simulink model "Control_Model"  (R2015a)
settings: Solver=ode1  StartTime=0.0  StopTime=150  FixedStep=0.002  MaxStep=0.01  MinStep=0.01  RelTol=1e-3
settings Model: Creator=Callum  LastModifiedBy=Callum
settings SolverCC: InitialStep=0.01
settings HardwareCC: TargetLongLongMode=on  TargetIntDivRoundTo=Zero  TargetEndianess=LittleEndian  TargetHWDeviceType=MATLAB Host  ProdEqTarget=off
settings RTWCC: SystemTargetFile=rsim.tlc  TemplateMakefile=rsim_default_tmf  Description=Rapid Simulation Target
settings RSimTargetCC: ERTMultiwordTypeDef=System defined  ERTMultiwordLength=256

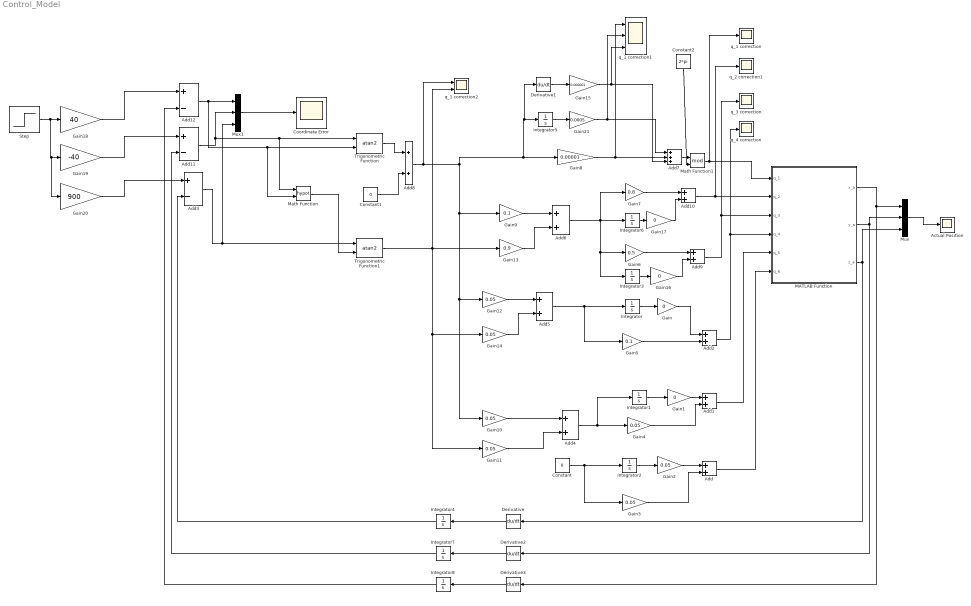
== system Control_Model ==
  Actual Position : Scope
      settings: YMin=-400  YMax=1200
  Add{,1..2,4..6,8..10} (9 alike) : Sum
  Add11 : Sum  Inputs=+-
  Add12 : Sum  Inputs=+-
  Add3 : Sum  Inputs=+-
  Add7 : Sum  Inputs=+++
  Constant : Constant  Value=0
  Constant1 : Constant  Value=0
  Constant2 : Constant  Value=2*pi
  Coordinate Error : Scope
      settings: SaveName=ScopeData7
  Derivative{,1..3} (4 alike) : Derivative
  Gain{,1,16..17} (4 alike) : Gain  Gain=0
  Gain{2..4,10..12,14} (7 alike) : Gain  Gain=0.05
  Gain13 : Gain  Gain=0.9
  Gain15 : Gain  Gain=0.000001
  Gain18 : Gain  Gain=40
  Gain19 : Gain  Gain=-40
  Gain20 : Gain  Gain=900
  Gain21 : Gain  Gain=0.0005
  Gain5 : Gain  Gain=0.1
  Gain6 : Gain  Gain=0.5
  Gain7 : Gain  Gain=0.8
  Gain8 : Gain  Gain=0.00001
  Gain9 : Gain  Gain=0.1
  Integrator{,1..8} (9 alike) : Integrator
  MATLAB Function : MATLAB Function  TreatAsAtomicUnit=on
  Math Function : Math  Operator=hypot  SaturateOnIntegerOverflow=on
  Math Function1 : Math  Operator=mod  SaturateOnIntegerOverflow=on
  Mux : Mux  Inputs=3
  Mux1 : Mux  Inputs=3
  Step : Step  SampleTime=0
  Trigonometric Function : Trigonometry  Operator=atan2
  Trigonometric Function1 : Trigonometry  Operator=atan2
  q_1 correction : Scope
      settings: YMin=0  YMax=6.5
  q_1 correction1 : Scope  NumInputPorts=3
      settings: YMin=-5~-5~-5  YMax=5~5~5  SaveName=ScopeData5
  q_1 correction2 : Scope  NumInputPorts=2
      settings: YMin=-5~-5  YMax=5~5  SaveName=ScopeData6
  q_2 correction1 : Scope
      settings: SaveName=ScopeData2
  q_3 correction : Scope
      settings: SaveName=ScopeData3
  q_4 correction : Scope
      settings: SaveName=ScopeData4
  wires:
  Integrator/1 -> Gain/1
  Integrator1/1 -> Gain1/1
  Integrator2/1 -> Gain2/1
  Constant/1 -> Integrator2/1, Gain3/1
  Gain2/1 -> Add/1
  Gain3/1 -> Add/2
  Add/1 -> MATLAB Function/6(q_6)
  Gain1/1 -> Add1/1
  Add1/1 -> MATLAB Function/5(q_5)
  Gain4/1 -> Add1/2
  Add2/1 -> q_4 correction/1, MATLAB Function/4(q_4)
  Gain/1 -> Add2/1
  Gain5/1 -> Add2/2
  Add4/1 -> Integrator1/1, Gain4/1
  Add5/1 -> Gain5/1, Integrator/1
  Add6/1 -> Gain6/1, Integrator3/1, Integrator6/1, Gain7/1
  Gain18/1 -> Add12/1
  Gain20/1 -> Add3/1
  Add11/1 -> Mux1/2, Math Function/1, Trigonometric Function/1
  MATLAB Function/1(x_a) -> Mux/1, Derivative3/1
  MATLAB Function/3(z_a) -> Mux/3, Derivative/1
  Gain10/1 -> Add4/1
  Gain11/1 -> Add4/2
  Gain14/1 -> Add5/2
  Add12/1 -> Mux1/1, Trigonometric Function/2, Math Function/2
  Step/1 -> Gain20/1, Gain19/1, Gain18/1
  Gain19/1 -> Add11/1
  Gain6/1 -> Add9/1
  Integrator4/1 -> Add3/2
  Derivative/1 -> Integrator4/1
  Integrator5/1 -> Gain21/1
  Gain21/1 -> q_1 correction1/2, Add7/1
  Add7/1 -> Math Function1/1
  Gain8/1 -> q_1 correction1/1, Add7/2
  Trigonometric Function/1 -> Add8/1
  Constant1/1 -> Add8/2
  Add8/1 -> q_1 correction2/1, Gain9/1, Gain10/1, Gain12/1, Derivative1/1, Integrator5/1, Gain8/1
  Gain12/1 -> Add5/1
  Gain13/1 -> Add6/2
  Gain9/1 -> Add6/1
  Trigonometric Function1/1 -> Gain13/1, q_1 correction2/2, Gain11/1, Gain14/1
  Add3/1 -> Mux1/3, Trigonometric Function1/1
  Math Function/1 -> Trigonometric Function1/2
  Derivative1/1 -> Gain15/1
  Gain15/1 -> q_1 correction1/3, Add7/3
  Math Function1/1 -> q_1 correction/1, MATLAB Function/1(q_1)
  Constant2/1 -> Math Function1/2
  Integrator3/1 -> Gain16/1
  Gain16/1 -> Add9/2
  Add9/1 -> q_3 correction/1, MATLAB Function/3(q_3)
  Integrator6/1 -> Gain17/1
  Gain7/1 -> Add10/1
  Gain17/1 -> Add10/2
  Add10/1 -> MATLAB Function/2(q_2), q_2 correction1/1
  MATLAB Function/2(y_a) -> Derivative2/1, Mux/2
  Integrator7/1 -> Add11/2
  Derivative2/1 -> Integrator7/1
  Derivative3/1 -> Integrator8/1
  Integrator8/1 -> Add12/2
  Mux/1 -> Actual Position/1
  Mux1/1 -> Coordinate Error/1

== matlab function Control_Model/MATLAB Function ==
  data: q_1 input; x_a output; q_2 input; q_3 input; q_4 input; q_5 input; q_6 input; y_a output; z_a output
function [x_a, y_a, z_a] = fcn(q_1, q_2, q_3, q_4, q_5, q_6)
%#codegen

q1 = q_1; %pi-(q_1);
q2 = q_2; %-pi/2 + (q_2+pi);
q3 = q_3; %pi/2 + (pi+q_3);
q4 = q_4; %q_4;
q5 = q_5; %-pi + q_5;
q6 = q_6; %pi + q_6;

%A_new = vpa(subs(A, [q1,q2,q3,q4,q5,q6], [ pi-(q_1), -pi/2 + (q_2+pi), pi/2 + (pi+q_3), q_4, -pi + q_5, pi]));


x_a = 9.8*sin(q1) + 410.0*cos(q1)*cos(q2) - 161.90703230275506147226218323136*cos(q4)*sin(q1) + 175.614064605510166451876962007*sin(q5)*(1.0*sin(q1)*sin(q4) - cos(q4)*(cos(q1)*cos(q2)*cos(q3) + cos(q1)*sin(q2)*sin(q3))) - 161.90703230275506147226218323136*sin(q4)*(cos(q1)*cos(q2)*cos(q3) + cos(q1)*sin(q2)*sin(q3)) - 175.614064605510166451876962007*cos(q5)*(0.5*cos(q4)*sin(q1) + 0.5*sin(q4)*(cos(q1)*cos(q2)*cos(q3) + cos(q1)*sin(q2)*sin(q3)) - 0.86602540378443864676372317075294*cos(q1)*cos(q2)*sin(q3) + 0.86602540378443864676372317075294*cos(q1)*cos(q3)*sin(q2)) - 343.55872363064032981583295622841*cos(q1)*cos(q2)*sin(q3) + 343.55872363064032981583295622841*cos(q1)*cos(q3)*sin(q2); 
y_a = 161.90703230275506147226218323136*cos(q1)*cos(q4) - 9.8*cos(q1) + 410.0*cos(q2)*sin(q1) + 175.614064605510166451876962007*cos(q5)*(0.5*cos(q1)*cos(q4) - 0.5*sin(q4)*(sin(q1)*sin(q2)*sin(q3) + cos(q2)*cos(q3)*sin(q1)) + 0.86602540378443864676372317075294*cos(q2)*sin(q1)*sin(q3) - 0.86602540378443864676372317075294*cos(q3)*sin(q1)*sin(q2)) - 175.614064605510166451876962007*sin(q5)*(1.0*cos(q1)*sin(q4) + cos(q4)*(sin(q1)*sin(q2)*sin(q3) + cos(q2)*cos(q3)*sin(q1))) - 161.90703230275506147226218323136*sin(q4)*(sin(q1)*sin(q2)*sin(q3) + cos(q2)*cos(q3)*sin(q1)) - 343.55872363064032981583295622841*cos(q2)*sin(q1)*sin(q3) + 343.55872363064032981583295622841*cos(q3)*sin(q1)*sin(q2);
z_a = 410.0*sin(q2) - 343.55872363064032981583295622841*cos(q2)*cos(q3) - 343.55872363064032981583295622841*sin(q2)*sin(q3) + 175.614064605510166451876962007*cos(q5)*(0.86602540378443864676372317075294*cos(q2)*cos(q3) + 0.86602540378443864676372317075294*sin(q2)*sin(q3) + 0.5*sin(q4)*(1.0*cos(q2)*sin(q3) - 1.0*cos(q3)*sin(q2))) + 161.90703230275506147226218323136*sin(q4)*(1.0*cos(q2)*sin(q3) - 1.0*cos(q3)*sin(q2)) + 175.614064605510166451876962007*cos(q4)*sin(q5)*(1.0*cos(q2)*sin(q3) - 1.0*cos(q3)*sin(q2)) + 197.13;




%y = u;
